simulink model "FOUR_WING"  (R2017a)
settings: Solver=VariableStepAuto  StartTime=0.0  StopTime=500  RelTol=1e-3
values from neighbouring files (symbols this model uses):
  a = 0.2    [PARAMETROS_FOUR_WING.m]
  b = -0.01    [PARAMETROS_FOUR_WING.m]
  c = 1    [PARAMETROS_FOUR_WING.m]
  d = -0.4    [PARAMETROS_FOUR_WING.m]
  f = -1.0    (= -1)    [PARAMETROS_FOUR_WING.m]
libraries: simulink x1
settings Model: Creator=Cesar  LastModifiedBy=Cesar

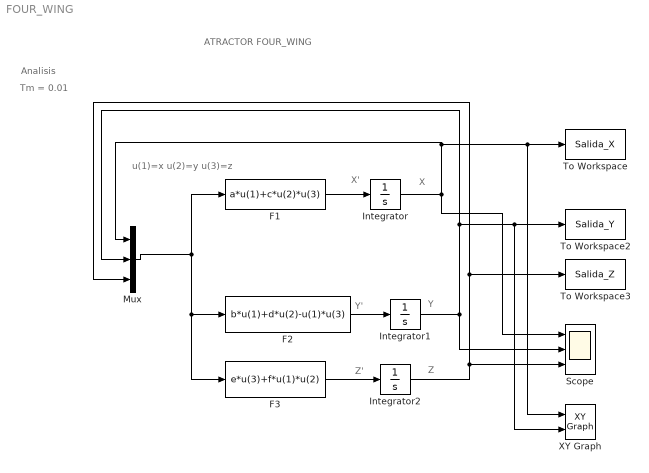
== system FOUR_WING ==
  note: Z
  note: Z'
  note: Analisis
  note: Tm = 0.01
  note: u(1)=x
      | u(2)=y
      | u(3)=z
  note: ATRACTOR FOUR_WING
  note: Y
  note: Y'
  note: X
  note: X'
  F1 : Fcn  Expr=a*u(1)+c*u(2)*u(3)
  F2 : Fcn  Expr=b*u(1)+d*u(2)-u(1)*u(3)
  F3 : Fcn  Expr=e*u(3)+f*u(1)*u(2)
  Integrator : Integrator  InitialCondition=0.5
  Integrator1 : Integrator  InitialCondition=0.5
  Integrator2 : Integrator  InitialCondition=0.5
  Mux : Mux  Inputs=3
  Scope : Scope  NumInputPorts=3
  To Workspace : ToWorkspace  VariableName=Salida_X  SampleTime=0.01
  To Workspace2 : ToWorkspace  VariableName=Salida_Y  SampleTime=0.01
  To Workspace3 : ToWorkspace  VariableName=Salida_Z  SampleTime=0.01
  XY Graph : simulink/Sinks/XY Graph  xmin=-5  xmax=5  ymin=-5  ymax=5  st=-1
  wires:
  F2/1 -> Integrator1/1
  F1/1 -> Integrator/1
  Mux/1 -> F1/1, F3/1, F2/1
  F3/1 -> Integrator2/1
  Integrator2/1 -> To Workspace3/1, Mux/3, Scope/3
  Integrator/1 -> Scope/1, XY Graph/1, To Workspace/1, Mux/1
  Integrator1/1 -> Scope/2, XY Graph/2, To Workspace2/1, Mux/2
